simulink model "Bodies_8_Lift_Actuation"  (R2024a)
settings: Solver=ode15s  StartTime=0.0  StopTime=10.0  MaxStep=1e-2  RelTol=1e-3  AbsTol=1e-4  EnableMultiTasking=on
PostLoadFcn:
  | warning off mech2:compiler:topologyAnalysis:DanglingBlock
values from neighbouring files (symbols this model uses):
  rad = 5    [Plot_Extr_Data_Ring_withBoxFillet_forSlide.m]    (also in Plot_Link_Extr_Data_forSlide.m)
undefined symbols (not defined in the file or in its folder): Local, SCL_Par, X, Y, Z
libraries: sm_lib x89, sm_scissor_lift_lib x28, nesl_utility x14, fl_lib x8, sh_lib x4, simulink x1
(part 2 of 4)

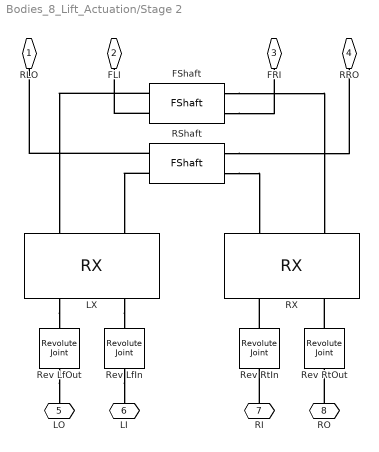
== system Bodies_8_Lift_Actuation/Stage 2 ==
  FShaft : sm_scissor_lift_lib/FShaft  sep_outer_outer=SCL_Par.Link_Sep.Outer_Outer  sep_outer_inner=SCL_Par.Link_Sep.Outer_Inner  shaft_radius=SCL_Par.Trans_Shaft.Radius  shaft_density=SCL_Par.Trans_Shaft.Density  shaft_color=SCL_Par.Trans_Shaft.Color  shaft_opacity=SCL_Par.Trans_Shaft.Opacity
  LX : sm_scissor_lift_lib/RX  leftright=Left  link_length_in=SCL_Par.Link.Length  link_length_out=SCL_Par.Link.Length  link_width_in=SCL_Par.Link.Width  link_width_out=SCL_Par.Link.Width  link_thickness_in=SCL_Par.Link.Thick  link_thickness_out=SCL_Par.Link.Thick  link_hole_radius_in=SCL_Par.Link.HolRad  link_hole_radius_out=SCL_Par.Link.HolRad  link_density_in=SCL_Par.Link.Density  link_density_out=SCL_Par.Link.Density  link_color_in=SCL_Par.Link.ColorI  link_color_out=SCL_Par.Link.ColorO  link_opacity_in=SCL_Par.Link.Opacity  link_opacity_out=SCL_Par.Link.Opacity  shaft_length=SCL_Par.Link_Sep.Outer_Inner  shaft_radius=SCL_Par.Link_Pin.Radius  shaft_density=SCL_Par.Link_Pin.Density  shaft_color=SCL_Par.Link_Pin.Color  shaft_opacity=SCL_Par.Link_Pin.Opacity  imgfile=Crossbar_RX_IMAGE.jpg
  RShaft : sm_scissor_lift_lib/FShaft  sep_outer_outer=SCL_Par.Link_Sep.Outer_Outer  sep_outer_inner=SCL_Par.Link_Sep.Outer_Inner  shaft_radius=SCL_Par.Trans_Shaft.Radius  shaft_density=SCL_Par.Trans_Shaft.Density  shaft_color=SCL_Par.Trans_Shaft.Color  shaft_opacity=SCL_Par.Trans_Shaft.Opacity
  RX : sm_scissor_lift_lib/RX  leftright=Right  link_length_in=SCL_Par.Link.Length  link_length_out=SCL_Par.Link.Length  link_width_in=SCL_Par.Link.Width  link_width_out=SCL_Par.Link.Width  link_thickness_in=SCL_Par.Link.Thick  link_thickness_out=SCL_Par.Link.Thick  link_hole_radius_in=SCL_Par.Link.HolRad  link_hole_radius_out=SCL_Par.Link.HolRad  link_density_in=SCL_Par.Link.Density  link_density_out=SCL_Par.Link.Density  link_color_in=SCL_Par.Link.ColorI  link_color_out=SCL_Par.Link.ColorO  link_opacity_in=SCL_Par.Link.Opacity  link_opacity_out=SCL_Par.Link.Opacity  shaft_length=SCL_Par.Link_Sep.Outer_Inner  shaft_radius=SCL_Par.Link_Pin.Radius  shaft_density=SCL_Par.Link_Pin.Density  shaft_color=SCL_Par.Link_Pin.Color  shaft_opacity=SCL_Par.Link_Pin.Opacity  imgfile=Crossbar_RX_IMAGE.jpg
  Rev LfIn : sm_lib/Joints/Revolute Joint  JointMode=Normal  CompositeWrenchDir=FollowerOnBase  CompositeWrenchFrame=BaseFrame  SenseConstraintForce=off  SenseConstraintTorque=off  SenseTotalForce=off  SenseTotalTorque=off  PositionTargetSpecify=off  PositionTargetPriority=Low  PositionTargetValue=0  PositionTargetValueUnits=deg  VelocityTargetSpecify=off  VelocityTargetPriority=High  VelocityTargetValue=0  VelocityTargetValueUnits=rad/s  EquilibriumPosition=0  EquilibriumPositionUnits=deg  SpringStiffness=0  SpringStiffnessUnits=N*m/rad  DampingCoefficient=0  DampingCoefficientUnits=N*m/(rad/s)  LowerLimitSpecify=off  LowerLimitBound=-90  LowerLimitBoundUnits=deg  LowerLimitStiffness=1e4  LowerLimitStiffnessUnits=N*m/deg  LowerLimitDamping=10  LowerLimitDampingUnits=N*m/(deg/s)  LowerLimitTransitionRegionWidth=0.1  LowerLimitTransitionRegionWidthUnits=deg  UpperLimitSpecify=off  UpperLimitBound=90  UpperLimitBoundUnits=deg  UpperLimitStiffness=1e4  UpperLimitStiffnessUnits=N*m/deg  UpperLimitDamping=10  UpperLimitDampingUnits=N*m/(deg/s)  UpperLimitTransitionRegionWidth=0.1  UpperLimitTransitionRegionWidthUnits=deg  TorqueActuationMode=NoTorque  MotionActuationMode=ComputedMotion  SensePosition=off  SenseVelocity=off  SenseAcceleration=off  SenseTorqueForce=off  SenseLowerLimitTorqueForce=off  SenseUpperLimitTorqueForce=off
  Rev LfOut : sm_lib/Joints/Revolute Joint  JointMode=Normal  CompositeWrenchDir=FollowerOnBase  CompositeWrenchFrame=BaseFrame  SenseConstraintForce=off  SenseConstraintTorque=off  SenseTotalForce=off  SenseTotalTorque=off  PositionTargetSpecify=off  PositionTargetPriority=Low  PositionTargetValue=0  PositionTargetValueUnits=deg  VelocityTargetSpecify=off  VelocityTargetPriority=High  VelocityTargetValue=0  VelocityTargetValueUnits=rad/s  EquilibriumPosition=0  EquilibriumPositionUnits=deg  SpringStiffness=0  SpringStiffnessUnits=N*m/rad  DampingCoefficient=0  DampingCoefficientUnits=N*m/(rad/s)  LowerLimitSpecify=off  LowerLimitBound=-90  LowerLimitBoundUnits=deg  LowerLimitStiffness=1e4  LowerLimitStiffnessUnits=N*m/deg  LowerLimitDamping=10  LowerLimitDampingUnits=N*m/(deg/s)  LowerLimitTransitionRegionWidth=0.1  LowerLimitTransitionRegionWidthUnits=deg  UpperLimitSpecify=off  UpperLimitBound=90  UpperLimitBoundUnits=deg  UpperLimitStiffness=1e4  UpperLimitStiffnessUnits=N*m/deg  UpperLimitDamping=10  UpperLimitDampingUnits=N*m/(deg/s)  UpperLimitTransitionRegionWidth=0.1  UpperLimitTransitionRegionWidthUnits=deg  TorqueActuationMode=NoTorque  MotionActuationMode=ComputedMotion  SensePosition=off  SenseVelocity=off  SenseAcceleration=off  SenseTorqueForce=off  SenseLowerLimitTorqueForce=off  SenseUpperLimitTorqueForce=off
  Rev RtIn : sm_lib/Joints/Revolute Joint  JointMode=Normal  CompositeWrenchDir=FollowerOnBase  CompositeWrenchFrame=BaseFrame  SenseConstraintForce=off  SenseConstraintTorque=off  SenseTotalForce=off  SenseTotalTorque=off  PositionTargetSpecify=on  PositionTargetPriority=High  PositionTargetValue=-2*SCL_Par.Init.Base_Angle  PositionTargetValueUnits=deg  VelocityTargetSpecify=off  VelocityTargetPriority=High  VelocityTargetValue=0  VelocityTargetValueUnits=rad/s  EquilibriumPosition=0  EquilibriumPositionUnits=deg  SpringStiffness=0  SpringStiffnessUnits=N*m/rad  DampingCoefficient=0  DampingCoefficientUnits=N*m/(rad/s)  LowerLimitSpecify=off  LowerLimitBound=-90  LowerLimitBoundUnits=deg  LowerLimitStiffness=1e4  LowerLimitStiffnessUnits=N*m/deg  LowerLimitDamping=10  LowerLimitDampingUnits=N*m/(deg/s)  LowerLimitTransitionRegionWidth=0.1  LowerLimitTransitionRegionWidthUnits=deg  UpperLimitSpecify=off  UpperLimitBound=90  UpperLimitBoundUnits=deg  UpperLimitStiffness=1e4  UpperLimitStiffnessUnits=N*m/deg  UpperLimitDamping=10  UpperLimitDampingUnits=N*m/(deg/s)  UpperLimitTransitionRegionWidth=0.1  UpperLimitTransitionRegionWidthUnits=deg  TorqueActuationMode=NoTorque  MotionActuationMode=ComputedMotion  SensePosition=off  SenseVelocity=off  SenseAcceleration=off  SenseTorqueForce=off  SenseLowerLimitTorqueForce=off  SenseUpperLimitTorqueForce=off
  Rev RtOut : sm_lib/Joints/Revolute Joint  JointMode=Normal  CompositeWrenchDir=FollowerOnBase  CompositeWrenchFrame=BaseFrame  SenseConstraintForce=off  SenseConstraintTorque=off  SenseTotalForce=off  SenseTotalTorque=off  PositionTargetSpecify=off  PositionTargetPriority=Low  PositionTargetValue=0  PositionTargetValueUnits=deg  VelocityTargetSpecify=off  VelocityTargetPriority=High  VelocityTargetValue=0  VelocityTargetValueUnits=rad/s  EquilibriumPosition=0  EquilibriumPositionUnits=deg  SpringStiffness=0  SpringStiffnessUnits=N*m/rad  DampingCoefficient=0  DampingCoefficientUnits=N*m/(rad/s)  LowerLimitSpecify=off  LowerLimitBound=-90  LowerLimitBoundUnits=deg  LowerLimitStiffness=1e4  LowerLimitStiffnessUnits=N*m/deg  LowerLimitDamping=10  LowerLimitDampingUnits=N*m/(deg/s)  LowerLimitTransitionRegionWidth=0.1  LowerLimitTransitionRegionWidthUnits=deg  UpperLimitSpecify=off  UpperLimitBound=90  UpperLimitBoundUnits=deg  UpperLimitStiffness=1e4  UpperLimitStiffnessUnits=N*m/deg  UpperLimitDamping=10  UpperLimitDampingUnits=N*m/(deg/s)  UpperLimitTransitionRegionWidth=0.1  UpperLimitTransitionRegionWidthUnits=deg  TorqueActuationMode=NoTorque  MotionActuationMode=ComputedMotion  SensePosition=off  SenseVelocity=off  SenseAcceleration=off  SenseTorqueForce=off  SenseLowerLimitTorqueForce=off  SenseUpperLimitTorqueForce=off
  RLO : PMIOPort  Side=Left
  FLI : PMIOPort  Port=2  Side=Left
  FRI : PMIOPort  Port=3  Side=Left
  RRO : PMIOPort  Port=4  Side=Left
  LO : PMIOPort  Port=5  Side=Right
  LI : PMIOPort  Port=6  Side=Right
  RI : PMIOPort  Port=7  Side=Right
  RO : PMIOPort  Port=8  Side=Right
  connections:
  Rev LfIn/LConn1 -- LI/RConn1
  Rev LfOut/LConn1 -- LO/RConn1
  LX/RConn2 -- Rev LfIn/RConn1
  LX/RConn1 -- Rev LfOut/RConn1
  RShaft/LConn2 -- LX/LConn2
  RShaft/LConn1 -- RLO/RConn1
  RShaft/RConn1 -- RRO/RConn1
  FShaft/LConn2 -- FLI/RConn1
  FShaft/LConn1 -- LX/LConn1
  FShaft/RConn2 -- FRI/RConn1
  RShaft/RConn2 -- RX/LConn1
  FShaft/RConn1 -- RX/LConn2
  Rev RtIn/RConn1 -- RX/RConn1
  Rev RtOut/RConn1 -- RX/RConn2
  RI/RConn1 -- Rev RtIn/LConn1
  RO/RConn1 -- Rev RtOut/LConn1

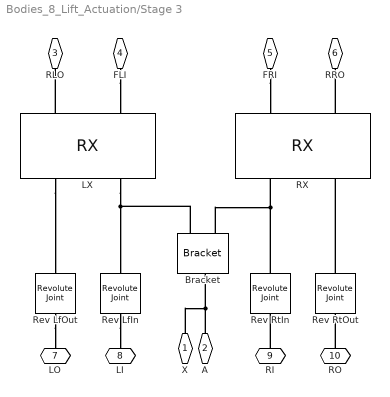
== system Bodies_8_Lift_Actuation/Stage 3 ==
  Bracket : sm_scissor_lift_lib/Bracket  fl_w=SCL_Par.Act.Brkt.Flange.Width  fl_h=SCL_Par.Act.Brkt.Flange.Height  T=SCL_Par.Act.Brkt.Flange.Thickness  w_link=SCL_Par.Link.Width  offset_l=SCL_Par.Act.Brkt.Flange.Offset_L  offset_h=SCL_Par.Act.Brkt.Flange.Offset_H  flupdown=Up  flfrontrear=Front  fl_density=SCL_Par.Act.Brkt.Flange.Density  fl_clr=SCL_Par.Act.Brkt.Flange.Color  fl_opc=SCL_Par.Act.Brkt.Flange.Opacity  shaft_length=SCL_Par.Link_Sep.Outer_Outer-SCL_Par.Link_Sep.Outer_Inner*2  shaft_radius=SCL_Par.Act.Brkt.Shaft.Radius  shaft_density=SCL_Par.Act.Brkt.Shaft.Density  shaft_color=SCL_Par.Act.Brkt.Shaft.Color  shaft_opacity=SCL_Par.Act.Brkt.Shaft.Opacity
  LX : sm_scissor_lift_lib/RX  leftright=Left  link_length_in=SCL_Par.Link.Length  link_length_out=SCL_Par.Link.Length  link_width_in=SCL_Par.Link.Width  link_width_out=SCL_Par.Link.Width  link_thickness_in=SCL_Par.Link.Thick  link_thickness_out=SCL_Par.Link.Thick  link_hole_radius_in=SCL_Par.Link.HolRad  link_hole_radius_out=SCL_Par.Link.HolRad  link_density_in=SCL_Par.Link.Density  link_density_out=SCL_Par.Link.Density  link_color_in=SCL_Par.Link.ColorI  link_color_out=SCL_Par.Link.ColorO  link_opacity_in=SCL_Par.Link.Opacity  link_opacity_out=SCL_Par.Link.Opacity  shaft_length=SCL_Par.Link_Sep.Outer_Inner  shaft_radius=SCL_Par.Link_Pin.Radius  shaft_density=SCL_Par.Link_Pin.Density  shaft_color=SCL_Par.Link_Pin.Color  shaft_opacity=SCL_Par.Link_Pin.Opacity  imgfile=Crossbar_RX_IMAGE.jpg
  RX : sm_scissor_lift_lib/RX  leftright=Right  link_length_in=SCL_Par.Link.Length  link_length_out=SCL_Par.Link.Length  link_width_in=SCL_Par.Link.Width  link_width_out=SCL_Par.Link.Width  link_thickness_in=SCL_Par.Link.Thick  link_thickness_out=SCL_Par.Link.Thick  link_hole_radius_in=SCL_Par.Link.HolRad  link_hole_radius_out=SCL_Par.Link.HolRad  link_density_in=SCL_Par.Link.Density  link_density_out=SCL_Par.Link.Density  link_color_in=SCL_Par.Link.ColorI  link_color_out=SCL_Par.Link.ColorO  link_opacity_in=SCL_Par.Link.Opacity  link_opacity_out=SCL_Par.Link.Opacity  shaft_length=SCL_Par.Link_Sep.Outer_Inner  shaft_radius=SCL_Par.Link_Pin.Radius  shaft_density=SCL_Par.Link_Pin.Density  shaft_color=SCL_Par.Link_Pin.Color  shaft_opacity=SCL_Par.Link_Pin.Opacity  imgfile=Crossbar_RX_IMAGE.jpg
  Rev LfIn : sm_lib/Joints/Revolute Joint  JointMode=Normal  CompositeWrenchDir=FollowerOnBase  CompositeWrenchFrame=BaseFrame  SenseConstraintForce=off  SenseConstraintTorque=off  SenseTotalForce=off  SenseTotalTorque=off  PositionTargetSpecify=off  PositionTargetPriority=Low  PositionTargetValue=0  PositionTargetValueUnits=deg  VelocityTargetSpecify=off  VelocityTargetPriority=High  VelocityTargetValue=0  VelocityTargetValueUnits=rad/s  EquilibriumPosition=0  EquilibriumPositionUnits=deg  SpringStiffness=0  SpringStiffnessUnits=N*m/rad  DampingCoefficient=0  DampingCoefficientUnits=N*m/(rad/s)  LowerLimitSpecify=off  LowerLimitBound=-90  LowerLimitBoundUnits=deg  LowerLimitStiffness=1e4  LowerLimitStiffnessUnits=N*m/deg  LowerLimitDamping=10  LowerLimitDampingUnits=N*m/(deg/s)  LowerLimitTransitionRegionWidth=0.1  LowerLimitTransitionRegionWidthUnits=deg  UpperLimitSpecify=off  UpperLimitBound=90  UpperLimitBoundUnits=deg  UpperLimitStiffness=1e4  UpperLimitStiffnessUnits=N*m/deg  UpperLimitDamping=10  UpperLimitDampingUnits=N*m/(deg/s)  UpperLimitTransitionRegionWidth=0.1  UpperLimitTransitionRegionWidthUnits=deg  TorqueActuationMode=NoTorque  MotionActuationMode=ComputedMotion  SensePosition=off  SenseVelocity=off  SenseAcceleration=off  SenseTorqueForce=off  SenseLowerLimitTorqueForce=off  SenseUpperLimitTorqueForce=off
  Rev LfOut : sm_lib/Joints/Revolute Joint  JointMode=Normal  CompositeWrenchDir=FollowerOnBase  CompositeWrenchFrame=BaseFrame  SenseConstraintForce=off  SenseConstraintTorque=off  SenseTotalForce=off  SenseTotalTorque=off  PositionTargetSpecify=off  PositionTargetPriority=Low  PositionTargetValue=0  PositionTargetValueUnits=deg  VelocityTargetSpecify=off  VelocityTargetPriority=High  VelocityTargetValue=0  VelocityTargetValueUnits=rad/s  EquilibriumPosition=0  EquilibriumPositionUnits=deg  SpringStiffness=0  SpringStiffnessUnits=N*m/rad  DampingCoefficient=0  DampingCoefficientUnits=N*m/(rad/s)  LowerLimitSpecify=off  LowerLimitBound=-90  LowerLimitBoundUnits=deg  LowerLimitStiffness=1e4  LowerLimitStiffnessUnits=N*m/deg  LowerLimitDamping=10  LowerLimitDampingUnits=N*m/(deg/s)  LowerLimitTransitionRegionWidth=0.1  LowerLimitTransitionRegionWidthUnits=deg  UpperLimitSpecify=off  UpperLimitBound=90  UpperLimitBoundUnits=deg  UpperLimitStiffness=1e4  UpperLimitStiffnessUnits=N*m/deg  UpperLimitDamping=10  UpperLimitDampingUnits=N*m/(deg/s)  UpperLimitTransitionRegionWidth=0.1  UpperLimitTransitionRegionWidthUnits=deg  TorqueActuationMode=NoTorque  MotionActuationMode=ComputedMotion  SensePosition=off  SenseVelocity=off  SenseAcceleration=off  SenseTorqueForce=off  SenseLowerLimitTorqueForce=off  SenseUpperLimitTorqueForce=off
  Rev RtIn : sm_lib/Joints/Revolute Joint  JointMode=Normal  CompositeWrenchDir=FollowerOnBase  CompositeWrenchFrame=BaseFrame  SenseConstraintForce=off  SenseConstraintTorque=off  SenseTotalForce=off  SenseTotalTorque=off  PositionTargetSpecify=on  PositionTargetPriority=High  PositionTargetValue=-2*SCL_Par.Init.Base_Angle  PositionTargetValueUnits=deg  VelocityTargetSpecify=off  VelocityTargetPriority=High  VelocityTargetValue=0  VelocityTargetValueUnits=rad/s  EquilibriumPosition=0  EquilibriumPositionUnits=deg  SpringStiffness=0  SpringStiffnessUnits=N*m/rad  DampingCoefficient=0  DampingCoefficientUnits=N*m/(rad/s)  LowerLimitSpecify=off  LowerLimitBound=-90  LowerLimitBoundUnits=deg  LowerLimitStiffness=1e4  LowerLimitStiffnessUnits=N*m/deg  LowerLimitDamping=10  LowerLimitDampingUnits=N*m/(deg/s)  LowerLimitTransitionRegionWidth=0.1  LowerLimitTransitionRegionWidthUnits=deg  UpperLimitSpecify=off  UpperLimitBound=90  UpperLimitBoundUnits=deg  UpperLimitStiffness=1e4  UpperLimitStiffnessUnits=N*m/deg  UpperLimitDamping=10  UpperLimitDampingUnits=N*m/(deg/s)  UpperLimitTransitionRegionWidth=0.1  UpperLimitTransitionRegionWidthUnits=deg  TorqueActuationMode=NoTorque  MotionActuationMode=ComputedMotion  SensePosition=off  SenseVelocity=off  SenseAcceleration=off  SenseTorqueForce=off  SenseLowerLimitTorqueForce=off  SenseUpperLimitTorqueForce=off
  Rev RtOut : sm_lib/Joints/Revolute Joint  JointMode=Normal  CompositeWrenchDir=FollowerOnBase  CompositeWrenchFrame=BaseFrame  SenseConstraintForce=off  SenseConstraintTorque=off  SenseTotalForce=off  SenseTotalTorque=off  PositionTargetSpecify=off  PositionTargetPriority=Low  PositionTargetValue=0  PositionTargetValueUnits=deg  VelocityTargetSpecify=off  VelocityTargetPriority=High  VelocityTargetValue=0  VelocityTargetValueUnits=rad/s  EquilibriumPosition=0  EquilibriumPositionUnits=deg  SpringStiffness=0  SpringStiffnessUnits=N*m/rad  DampingCoefficient=0  DampingCoefficientUnits=N*m/(rad/s)  LowerLimitSpecify=off  LowerLimitBound=-90  LowerLimitBoundUnits=deg  LowerLimitStiffness=1e4  LowerLimitStiffnessUnits=N*m/deg  LowerLimitDamping=10  LowerLimitDampingUnits=N*m/(deg/s)  LowerLimitTransitionRegionWidth=0.1  LowerLimitTransitionRegionWidthUnits=deg  UpperLimitSpecify=off  UpperLimitBound=90  UpperLimitBoundUnits=deg  UpperLimitStiffness=1e4  UpperLimitStiffnessUnits=N*m/deg  UpperLimitDamping=10  UpperLimitDampingUnits=N*m/(deg/s)  UpperLimitTransitionRegionWidth=0.1  UpperLimitTransitionRegionWidthUnits=deg  TorqueActuationMode=NoTorque  MotionActuationMode=ComputedMotion  SensePosition=off  SenseVelocity=off  SenseAcceleration=off  SenseTorqueForce=off  SenseLowerLimitTorqueForce=off  SenseUpperLimitTorqueForce=off
  X : PMIOPort  Side=Left
  A : PMIOPort  Port=2  Side=Right
  RLO : PMIOPort  Port=3  Side=Left
  FLI : PMIOPort  Port=4  Side=Left
  FRI : PMIOPort  Port=5  Side=Left
  RRO : PMIOPort  Port=6  Side=Left
  LO : PMIOPort  Port=7  Side=Right
  LI : PMIOPort  Port=8  Side=Right
  RI : PMIOPort  Port=9  Side=Right
  RO : PMIOPort  Port=10  Side=Right
  connections:
  X/RConn1 -- Bracket/LConn1 -- A/RConn1
  Rev RtIn/RConn1 -- Bracket/RConn2 -- RX/RConn1
  RO/RConn1 -- Rev RtOut/LConn1
  RX/LConn2 -- RRO/RConn1
  FLI/RConn1 -- LX/LConn2
  Rev RtOut/RConn1 -- RX/RConn2
  LX/RConn2 -- Bracket/RConn1 -- Rev LfIn/RConn1
  Rev LfOut/LConn1 -- LO/RConn1
  RI/RConn1 -- Rev RtIn/LConn1
  LX/RConn1 -- Rev LfOut/RConn1
  Rev LfIn/LConn1 -- LI/RConn1
  LX/LConn1 -- RLO/RConn1
  FRI/RConn1 -- RX/LConn1

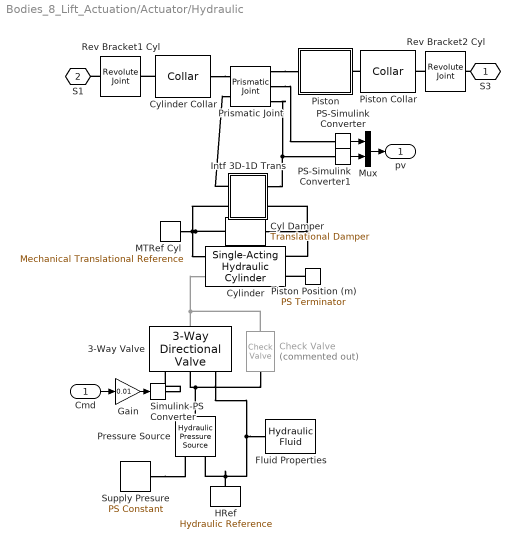
== system Bodies_8_Lift_Actuation/Actuator/Hydraulic ==
  Cmd : Inport
  3-Way Valve : sh_lib/Valves/Directional Valves/3-Way Directional Valve  Tag=Factory Generic  area_spec=1  mdl_type_identical=1  mdl_type_different=1  interp_method_identical=1  interp_method_different=1  extrap_method_identical=1  extrap_method_different=1  A_leak=1e-9 m^2  C_d=0.7  lam_spec=2  B_lam=0.999  Re_cr=12  opening_max=0.01 m  area_max=1e-4*0.1 m^2  opening_max_P_A=0.005 m  area_max_P_A=0.5e-4 m^2  opening_max_A_T=0.005 m  area_max_A_T=0.5e-4 m^2  opening_area_tab="[  -0.002 0 0.005 0.015 ] m"  area_tab="[  1e-12 4e-12 1e-05 1.02e-05 ] m^2"  opening_flow_rate_tab="[  -0.002 0 0.005 0.015 ] m"  pressure_tab="[  -5e+06 -2e+06 2e+06 5e+06 ] Pa"  flow_rate_tab="[  -1e-12 -6e-14 6e+12 1e+11 ; -8e-08 -4e-08 4e+06 8e+06 ; -0.0025 -0.00103 0.001 0.0024 ; -0.00258 -0.001032 0.00106 0.00247 ; ] m^3/s"  opening_area_tab_P_A=[-0.002, 0.0, 0.002, 0.005, 0.015] m  area_tab_P_A=[1.0e-9, 2.0352e-7, 4.0736e-5, 0.00011438, 0.00034356] m^2  opening_flow_rate_tab_P_A=[-0.002, 0.0, 0.002, 0.005, 0.015] m  pressure_tab_P_A=[-10000000.0, -5000000.0, -2000000.0, 2000000.0, 5000000.0, 10000000.0] Pa  flow_rate_tab_P_A=[-1.0e-7, -7.0711e-8, -4.4721e-8, 4.4721e-8, 7.0711e-8, 1.0e-7; -2.0352e-5, -1.4391e-5, -9.1017e-6, 9.1017e-6, 1.4391e-5, 2.0352e-5; -0.0040736, -0.0028805, -0.0018218, 0.0018218, 0.0028805, 0.0040736; -0.011438, -0.0080879, -0.0051152, 0.0051152, 0.0080879, 0.011438; -0.034356, -0.024293, -0.015364, 0.015364, 0.024293, 0.034356] m^3/s  opening_area_tab_A_T=[-0.002, 0.0, 0.002, 0.005, 0.015] m  area_tab_A_T=[1.0e-9, 2.0352e-7, 4.0736e-5, 0.00011438, 0.00034356] m^2  opening_flow_rate_tab_A_T=[-0.002, 0.0, 0.002, 0.005, 0.015] m  pressure_tab_A_T=[-10000000.0, -5000000.0, -2000000.0, 2000000.0, 5000000.0, 10000000.0] Pa  flow_rate_tab_A_T=[-1.0e-7, -7.0711e-8, -4.4721e-8, 4.4721e-8, 7.0711e-8, 1.0e-7; -2.0352e-5, -1.4391e-5, -9.1017e-6, 9.1017e-6, 1.4391e-5, 2.0352e-5; -0.0040736, -0.0028805, -0.0018218, 0.0018218, 0.0028805, 0.0040736; -0.011438, -0.0080879, -0.0051152, 0.0051152, 0.0080879, 0.011438; -0.034356, -0.024293, -0.015364, 0.015364, 0.024293, 0.034356] m^3/s  x_0_P=-0.008 m  x_0_T=-0.008 m
      settings: InternalSimscapePortConfiguration="{\"Bottom\":[],\"Left\":[{\"id\":\"A\",\"label\":\"A\",\"type\":\"foundation.hydraulic.hydraulic\"}],\"Right\":[{\"id\":\"S\",\"label\":\"S\",\"type\":\"input\"},{\"id\":\"P\",\"label\":\"P\",\"type\":\"foundation.hydraulic.hydraulic\"},{\"id\":\"T\",\"label\":\"T\",\"type\":\"foundation.hydraulic.hydraulic\"}],\"Top\":[]}"
  Check Valve : sh_lib/Valves/Directional Valves/Check Valve  Commented=on  area_max=1e-4 m^2  pres_crack=7e6 Pa  pres_max=7.2e6 Pa  C_d=0.7  A_leak=1e-12 m^2  lam_spec=2  B_lam=0.999  Re_cr=12  dynamic=0  tau=0.1 s  area_init=1e-12 m^2
      settings: InternalSimscapePortConfiguration="{\"Bottom\":[],\"Left\":[{\"id\":\"A\",\"label\":\"A\",\"type\":\"foundation.hydraulic.hydraulic\"}],\"Right\":[{\"id\":\"B\",\"label\":\"B\",\"type\":\"foundation.hydraulic.hydraulic\"}],\"Top\":[]}"
  Cyl Damper : fl_lib/Mechanical/Translational Elements/Translational Damper  D=SCL_Par.Act.Spring.Damping*4 N/(m/s)  v_specify=off  v_priority=None  v=0 m/s  v_nominal_specify=off  v_nominal_value=1  v_nominal_unit=m/s  f_specify=off  f_priority=None  f=0 N  f_nominal_specify=off  f_nominal_value=1  f_nominal_unit=N
  Cylinder : sh_lib/Hydraulic Cylinders/Single-Acting Hydraulic Cylinder  Tag=Factory Generic  area=0.002 m^2  stroke=2 m  displacement_spec=foundation.enum.DisplacementSpec.Calculate  init_pos=1 m  dead_vol=1e-06 m^3  init_pressure=0 Pa  k_sh=1.4  stiff=1e+07 N/m  D=250 N/(m/s)  hardstop_model=3  transition=0.1 mm  or=1
      settings: InternalSimscapePortConfiguration="{\"Bottom\":[],\"Left\":[{\"id\":\"C\",\"label\":\"C\",\"type\":\"foundation.mechanical.translational.translational\"},{\"id\":\"A\",\"label\":\"A\",\"type\":\"foundation.hydraulic.hydraulic\"}],\"Right\":[{\"id\":\"R\",\"label\":\"R\",\"type\":\"foundation.mechanical.translational.translational\"},{\"id\":\"P\",\"label\":\"p\",\"type\":\"output\"}],\"Top\":[]}"
  Cylinder Collar : sm_scissor_lift_lib/Collar  collar_length=SCL_Par.Act.Collar.Length  collar_radius=SCL_Par.Act.Collar.Radius  cylinder_length=SCL_Par.Act.Cylinder.Length  cylinder_radius=SCL_Par.Act.Cylinder.Radius  cylinder_ori=Local +Z  material_density=SCL_Par.Act.Collar.Density  material_color=SCL_Par.Act.Collar.Color  material_opacity=SCL_Par.Act.Collar.Opacity
  Fluid Properties : sh_lib/Hydraulic Utilities/Hydraulic Fluid  Tag=Factory Generic  SelFluid=1  SysTemp=40  TrapAir=0.002  ViscDerFactor=1  range_error=2
  Gain : Gain  Gain=0.01
  HRef : fl_lib/Hydraulic/Hydraulic Elements/Hydraulic Reference  Tag=Factory Generic
  Intf 3D-1D Trans : Subsystem
  MTRef Cyl : fl_lib/Mechanical/Translational Elements/Mechanical Translational Reference  Tag=Factory Generic
  Mux : Mux  Inputs=2
  PS-Simulink Converter : nesl_utility/PS-Simulink Converter  PhysicalDomain=network_engine_domain  SubClassName=ps_output  LeftPortType=input  RightPortType=output  PseudoPeriodic=off  Frequencies=[]  VectorFormat=1-D array  Unit=1  AffineConversion=off
  PS-Simulink Converter1 : nesl_utility/PS-Simulink Converter  PhysicalDomain=network_engine_domain  SubClassName=ps_output  LeftPortType=input  RightPortType=output  PseudoPeriodic=off  Frequencies=[]  VectorFormat=1-D array  Unit=1  AffineConversion=off
  Piston : Subsystem
      mask Display: image('Piston_Shaft_IMAGE.jpg');
  Piston Collar : sm_scissor_lift_lib/Collar  collar_length=SCL_Par.Act.Collar.Length  collar_radius=SCL_Par.Act.Collar.Radius  cylinder_length=SCL_Par.Act.Piston_Seat.Length  cylinder_radius=SCL_Par.Act.Piston_Seat.Radius  cylinder_ori=Local -Z  material_density=SCL_Par.Act.Collar.Density  material_color=SCL_Par.Act.Collar.Color  material_opacity=SCL_Par.Act.Collar.Opacity
  Piston Position (m) : fl_lib/Physical Signals/Sinks/PS Terminator
  Pressure Source : fl_lib/Hydraulic/Hydraulic Sources/Hydraulic Pressure Source  Tag=Factory Generic
      settings: InternalSimscapePortConfiguration="{\"Bottom\":[],\"Left\":[{\"id\":\"P\",\"label\":\"P\",\"type\":\"foundation.hydraulic.hydraulic\"}],\"Right\":[{\"id\":\"S\",\"label\":\"S\",\"type\":\"input\"},{\"id\":\"T\",\"label\":\"T\",\"type\":\"foundation.hydraulic.hydraulic\"}],\"Top\":[]}"
  Prismatic Joint : sm_lib/Joints/Prismatic Joint  JointMode=Normal  CompositeWrenchDir=FollowerOnBase  CompositeWrenchFrame=BaseFrame  SenseConstraintForce=off  SenseConstraintTorque=off  SenseTotalForce=off  SenseTotalTorque=off  PositionTargetSpecify=off  PositionTargetPriority=High  PositionTargetValue=0  PositionTargetValueUnits=m  VelocityTargetSpecify=off  VelocityTargetPriority=High  VelocityTargetValue=0  VelocityTargetValueUnits=m/s  EquilibriumPosition=SCL_Par.Act.Spring.Equilibrium_Position*0  EquilibriumPositionUnits=cm  SpringStiffness=SCL_Par.Act.Spring.Stiffness*0  SpringStiffnessUnits=N/m  DampingCoefficient=SCL_Par.Act.Spring.Damping*0  DampingCoefficientUnits=N/(m/s)  LowerLimitSpecify=off  LowerLimitBound=-1  LowerLimitBoundUnits=m  LowerLimitStiffness=1e6  LowerLimitStiffnessUnits=N/m  LowerLimitDamping=1e3  LowerLimitDampingUnits=N/(m/s)  LowerLimitTransitionRegionWidth=1e-4  LowerLimitTransitionRegionWidthUnits=m  UpperLimitSpecify=off  UpperLimitBound=1  UpperLimitBoundUnits=m  UpperLimitStiffness=1e6  UpperLimitStiffnessUnits=N/m  UpperLimitDamping=1e3  UpperLimitDampingUnits=N/(m/s)  UpperLimitTransitionRegionWidth=1e-4  UpperLimitTransitionRegionWidthUnits=m  TorqueActuationMode=InputTorque  MotionActuationMode=ComputedMotion  SensePosition=on  SenseVelocity=on  SenseAcceleration=off  SenseTorqueForce=off  SenseLowerLimitTorqueForce=off  SenseUpperLimitTorqueForce=off
  Rev Bracket1 Cyl : sm_lib/Joints/Revolute Joint  JointMode=Normal  CompositeWrenchDir=FollowerOnBase  CompositeWrenchFrame=BaseFrame  SenseConstraintForce=off  SenseConstraintTorque=off  SenseTotalForce=off  SenseTotalTorque=off  PositionTargetSpecify=off  PositionTargetPriority=High  PositionTargetValue=0  PositionTargetValueUnits=rad  VelocityTargetSpecify=off  VelocityTargetPriority=High  VelocityTargetValue=0  VelocityTargetValueUnits=rad/s  EquilibriumPosition=0  EquilibriumPositionUnits=rad  SpringStiffness=0  SpringStiffnessUnits=N*m/rad  DampingCoefficient=0  DampingCoefficientUnits=N*m/(rad/s)  LowerLimitSpecify=off  LowerLimitBound=-90  LowerLimitBoundUnits=deg  LowerLimitStiffness=1e4  LowerLimitStiffnessUnits=N*m/deg  LowerLimitDamping=10  LowerLimitDampingUnits=N*m/(deg/s)  LowerLimitTransitionRegionWidth=0.1  LowerLimitTransitionRegionWidthUnits=deg  UpperLimitSpecify=off  UpperLimitBound=90  UpperLimitBoundUnits=deg  UpperLimitStiffness=1e4  UpperLimitStiffnessUnits=N*m/deg  UpperLimitDamping=10  UpperLimitDampingUnits=N*m/(deg/s)  UpperLimitTransitionRegionWidth=0.1  UpperLimitTransitionRegionWidthUnits=deg  TorqueActuationMode=NoTorque  MotionActuationMode=ComputedMotion  SensePosition=off  SenseVelocity=off  SenseAcceleration=off  SenseTorqueForce=off  SenseLowerLimitTorqueForce=off  SenseUpperLimitTorqueForce=off
  Rev Bracket2 Cyl : sm_lib/Joints/Revolute Joint  JointMode=Normal  CompositeWrenchDir=FollowerOnBase  CompositeWrenchFrame=BaseFrame  SenseConstraintForce=off  SenseConstraintTorque=off  SenseTotalForce=off  SenseTotalTorque=off  PositionTargetSpecify=off  PositionTargetPriority=High  PositionTargetValue=0  PositionTargetValueUnits=rad  VelocityTargetSpecify=off  VelocityTargetPriority=High  VelocityTargetValue=0  VelocityTargetValueUnits=rad/s  EquilibriumPosition=0  EquilibriumPositionUnits=rad  SpringStiffness=0  SpringStiffnessUnits=N*m/rad  DampingCoefficient=0  DampingCoefficientUnits=N*m/(rad/s)  LowerLimitSpecify=off  LowerLimitBound=-90  LowerLimitBoundUnits=deg  LowerLimitStiffness=1e4  LowerLimitStiffnessUnits=N*m/deg  LowerLimitDamping=10  LowerLimitDampingUnits=N*m/(deg/s)  LowerLimitTransitionRegionWidth=0.1  LowerLimitTransitionRegionWidthUnits=deg  UpperLimitSpecify=off  UpperLimitBound=90  UpperLimitBoundUnits=deg  UpperLimitStiffness=1e4  UpperLimitStiffnessUnits=N*m/deg  UpperLimitDamping=10  UpperLimitDampingUnits=N*m/(deg/s)  UpperLimitTransitionRegionWidth=0.1  UpperLimitTransitionRegionWidthUnits=deg  TorqueActuationMode=NoTorque  MotionActuationMode=ComputedMotion  SensePosition=off  SenseVelocity=off  SenseAcceleration=off  SenseTorqueForce=off  SenseLowerLimitTorqueForce=off  SenseUpperLimitTorqueForce=off
  Simulink-PS Converter : nesl_utility/Simulink-PS Converter  PhysicalDomain=network_engine_domain  SubClassName=ps_input  LeftPortType=input  RightPortType=output  PseudoPeriodic=off  Frequencies=[]  NoiseDistribution=none  NoiseParameters=[]  Unit=m  AffineConversion=off  FilteringAndDerivatives=filter  SimscapeFilterOrder=1  InputFilterTimeConstant=0.005  UdotUserProvided=1
  Supply Presure : fl_lib/Physical Signals/Sources/PS Constant  constant=10e5*8
  S3 : PMIOPort  Side=Right
  S1 : PMIOPort  Port=2  Side=Left
  pv : Outport  VectorParamsAs1DForOutWhenUnconnected=off
  wires:
  Mux/1 -> pv/1
  PS-Simulink Converter1/1 -> Mux/2
  PS-Simulink Converter/1 -> Mux/1
  Cmd/1 -> Gain/1
  Gain/1 -> Simulink-PS Converter/1
  connections:
  Rev Bracket1 Cyl/LConn1 -- S1/RConn1
  S3/RConn1 -- Rev Bracket2 Cyl/LConn1
  Rev Bracket2 Cyl/RConn1 -- Piston Collar/LConn1
  Piston Collar/RConn1 -- Piston/LConn1
  Cylinder Collar/LConn1 -- Rev Bracket1 Cyl/RConn1
  Prismatic Joint/RConn1 -- Piston/RConn1
  Prismatic Joint/RConn2 -- PS-Simulink Converter/LConn1
  Prismatic Joint/RConn3 -- PS-Simulink Converter1/LConn1 -- Intf 3D-1D Trans/LConn1
  Cylinder Collar/RConn1 -- Prismatic Joint/LConn1
  Check Valve/RConn1 -- Cylinder/LConn2 -- 3-Way Valve/LConn1
  Cyl Damper/RConn1 -- MTRef Cyl/LConn1 -- Cylinder/LConn1 -- Intf 3D-1D Trans/RConn2
  3-Way Valve/RConn2 -- Pressure Source/LConn1 -- Check Valve/LConn1
  Intf 3D-1D Trans/LConn2 -- Cyl Damper/LConn1 -- Cylinder/RConn1
  Fluid Properties/RConn1 -- 3-Way Valve/RConn3 -- HRef/LConn1 -- Pressure Source/RConn2
  Simulink-PS Converter/RConn1 -- 3-Way Valve/RConn1
  Supply Presure/RConn1 -- Pressure Source/RConn1
  Piston Position (m)/LConn1 -- Cylinder/RConn2
  Intf 3D-1D Trans/RConn1 -- Prismatic Joint/LConn2

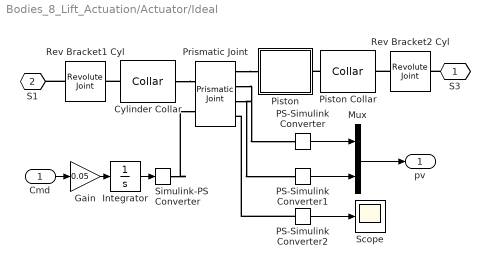
== system Bodies_8_Lift_Actuation/Actuator/Ideal ==
  Cmd : Inport
  Cylinder Collar : sm_scissor_lift_lib/Collar  collar_length=SCL_Par.Act.Collar.Length  collar_radius=SCL_Par.Act.Collar.Radius  cylinder_length=SCL_Par.Act.Cylinder.Length  cylinder_radius=SCL_Par.Act.Cylinder.Radius  cylinder_ori=Local +Z  material_density=SCL_Par.Act.Collar.Density  material_color=SCL_Par.Act.Collar.Color  material_opacity=SCL_Par.Act.Collar.Opacity
  Gain : Gain  Gain=0.05
  Integrator : Integrator  InitialCondition=1.89
  Mux : Mux  Inputs=2
  PS-Simulink Converter : nesl_utility/PS-Simulink Converter  PhysicalDomain=network_engine_domain  SubClassName=ps_output  LeftPortType=input  RightPortType=output  PseudoPeriodic=off  Frequencies=[]  VectorFormat=1-D array  Unit=1  AffineConversion=off
  PS-Simulink Converter1 : nesl_utility/PS-Simulink Converter  PhysicalDomain=network_engine_domain  SubClassName=ps_output  LeftPortType=input  RightPortType=output  PseudoPeriodic=off  Frequencies=[]  VectorFormat=1-D array  Unit=1  AffineConversion=off
  PS-Simulink Converter2 : nesl_utility/PS-Simulink Converter  PhysicalDomain=network_engine_domain  SubClassName=ps_output  LeftPortType=input  RightPortType=output  PseudoPeriodic=off  Frequencies=[]  VectorFormat=1-D array  Unit=1  AffineConversion=off
  Piston : Subsystem
      mask Display: image('Piston_Shaft_IMAGE.jpg');
  Piston Collar : sm_scissor_lift_lib/Collar  collar_length=SCL_Par.Act.Collar.Length  collar_radius=SCL_Par.Act.Collar.Radius  cylinder_length=SCL_Par.Act.Piston_Seat.Length  cylinder_radius=SCL_Par.Act.Piston_Seat.Radius  cylinder_ori=Local -Z  material_density=SCL_Par.Act.Collar.Density  material_color=SCL_Par.Act.Collar.Color  material_opacity=SCL_Par.Act.Collar.Opacity
  Prismatic Joint : sm_lib/Joints/Prismatic Joint  JointMode=Normal  CompositeWrenchDir=FollowerOnBase  CompositeWrenchFrame=BaseFrame  SenseConstraintForce=off  SenseConstraintTorque=off  SenseTotalForce=off  SenseTotalTorque=off  PositionTargetSpecify=off  PositionTargetPriority=High  PositionTargetValue=0  PositionTargetValueUnits=m  VelocityTargetSpecify=off  VelocityTargetPriority=High  VelocityTargetValue=0  VelocityTargetValueUnits=m/s  EquilibriumPosition=SCL_Par.Act.Spring.Equilibrium_Position  EquilibriumPositionUnits=cm  SpringStiffness=SCL_Par.Act.Spring.Stiffness  SpringStiffnessUnits=N/m  DampingCoefficient=SCL_Par.Act.Spring.Damping  DampingCoefficientUnits=N/(m/s)  LowerLimitSpecify=off  LowerLimitBound=-1  LowerLimitBoundUnits=m  LowerLimitStiffness=1e6  LowerLimitStiffnessUnits=N/m  LowerLimitDamping=1e3  LowerLimitDampingUnits=N/(m/s)  LowerLimitTransitionRegionWidth=1e-4  LowerLimitTransitionRegionWidthUnits=m  UpperLimitSpecify=off  UpperLimitBound=1  UpperLimitBoundUnits=m  UpperLimitStiffness=1e6  UpperLimitStiffnessUnits=N/m  UpperLimitDamping=1e3  UpperLimitDampingUnits=N/(m/s)  UpperLimitTransitionRegionWidth=1e-4  UpperLimitTransitionRegionWidthUnits=m  TorqueActuationMode=ComputedTorque  MotionActuationMode=InputMotion  SensePosition=on  SenseVelocity=on  SenseAcceleration=off  SenseTorqueForce=on  SenseLowerLimitTorqueForce=off  SenseUpperLimitTorqueForce=off
  Rev Bracket1 Cyl : sm_lib/Joints/Revolute Joint  JointMode=Normal  CompositeWrenchDir=FollowerOnBase  CompositeWrenchFrame=BaseFrame  SenseConstraintForce=off  SenseConstraintTorque=off  SenseTotalForce=off  SenseTotalTorque=off  PositionTargetSpecify=off  PositionTargetPriority=High  PositionTargetValue=0  PositionTargetValueUnits=rad  VelocityTargetSpecify=off  VelocityTargetPriority=High  VelocityTargetValue=0  VelocityTargetValueUnits=rad/s  EquilibriumPosition=0  EquilibriumPositionUnits=rad  SpringStiffness=0  SpringStiffnessUnits=N*m/rad  DampingCoefficient=0  DampingCoefficientUnits=N*m/(rad/s)  LowerLimitSpecify=off  LowerLimitBound=-90  LowerLimitBoundUnits=deg  LowerLimitStiffness=1e4  LowerLimitStiffnessUnits=N*m/deg  LowerLimitDamping=10  LowerLimitDampingUnits=N*m/(deg/s)  LowerLimitTransitionRegionWidth=0.1  LowerLimitTransitionRegionWidthUnits=deg  UpperLimitSpecify=off  UpperLimitBound=90  UpperLimitBoundUnits=deg  UpperLimitStiffness=1e4  UpperLimitStiffnessUnits=N*m/deg  UpperLimitDamping=10  UpperLimitDampingUnits=N*m/(deg/s)  UpperLimitTransitionRegionWidth=0.1  UpperLimitTransitionRegionWidthUnits=deg  TorqueActuationMode=NoTorque  MotionActuationMode=ComputedMotion  SensePosition=off  SenseVelocity=off  SenseAcceleration=off  SenseTorqueForce=off  SenseLowerLimitTorqueForce=off  SenseUpperLimitTorqueForce=off
  Rev Bracket2 Cyl : sm_lib/Joints/Revolute Joint  JointMode=Normal  CompositeWrenchDir=FollowerOnBase  CompositeWrenchFrame=BaseFrame  SenseConstraintForce=off  SenseConstraintTorque=off  SenseTotalForce=off  SenseTotalTorque=off  PositionTargetSpecify=off  PositionTargetPriority=High  PositionTargetValue=0  PositionTargetValueUnits=rad  VelocityTargetSpecify=off  VelocityTargetPriority=High  VelocityTargetValue=0  VelocityTargetValueUnits=rad/s  EquilibriumPosition=0  EquilibriumPositionUnits=rad  SpringStiffness=0  SpringStiffnessUnits=N*m/rad  DampingCoefficient=0  DampingCoefficientUnits=N*m/(rad/s)  LowerLimitSpecify=off  LowerLimitBound=-90  LowerLimitBoundUnits=deg  LowerLimitStiffness=1e4  LowerLimitStiffnessUnits=N*m/deg  LowerLimitDamping=10  LowerLimitDampingUnits=N*m/(deg/s)  LowerLimitTransitionRegionWidth=0.1  LowerLimitTransitionRegionWidthUnits=deg  UpperLimitSpecify=off  UpperLimitBound=90  UpperLimitBoundUnits=deg  UpperLimitStiffness=1e4  UpperLimitStiffnessUnits=N*m/deg  UpperLimitDamping=10  UpperLimitDampingUnits=N*m/(deg/s)  UpperLimitTransitionRegionWidth=0.1  UpperLimitTransitionRegionWidthUnits=deg  TorqueActuationMode=NoTorque  MotionActuationMode=ComputedMotion  SensePosition=off  SenseVelocity=off  SenseAcceleration=off  SenseTorqueForce=off  SenseLowerLimitTorqueForce=off  SenseUpperLimitTorqueForce=off
  Scope : Scope
  Simulink-PS Converter : nesl_utility/Simulink-PS Converter  PhysicalDomain=network_engine_domain  SubClassName=ps_input  LeftPortType=input  RightPortType=output  PseudoPeriodic=off  Frequencies=[]  NoiseDistribution=none  NoiseParameters=[]  Unit=1  AffineConversion=off  FilteringAndDerivatives=filter  SimscapeFilterOrder=2  InputFilterTimeConstant=0.005  UdotUserProvided=0
  S3 : PMIOPort  Side=Right
  S1 : PMIOPort  Port=2  Side=Left
  pv : Outport  VectorParamsAs1DForOutWhenUnconnected=off
  wires:
  PS-Simulink Converter/1 -> Mux/1
  PS-Simulink Converter1/1 -> Mux/2
  Mux/1 -> pv/1
  Gain/1 -> Integrator/1
  Cmd/1 -> Gain/1
  Integrator/1 -> Simulink-PS Converter/1
  PS-Simulink Converter2/1 -> Scope/1
  connections:
  Cylinder Collar/RConn1 -- Prismatic Joint/LConn1
  Prismatic Joint/RConn3 -- PS-Simulink Converter1/LConn1
  Prismatic Joint/RConn2 -- PS-Simulink Converter/LConn1
  Prismatic Joint/RConn1 -- Piston/RConn1
  Cylinder Collar/LConn1 -- Rev Bracket1 Cyl/RConn1
  Piston Collar/RConn1 -- Piston/LConn1
  Rev Bracket2 Cyl/RConn1 -- Piston Collar/LConn1
  S3/RConn1 -- Rev Bracket2 Cyl/LConn1
  Rev Bracket1 Cyl/LConn1 -- S1/RConn1
  Simulink-PS Converter/RConn1 -- Prismatic Joint/LConn2
  PS-Simulink Converter2/LConn1 -- Prismatic Joint/RConn4

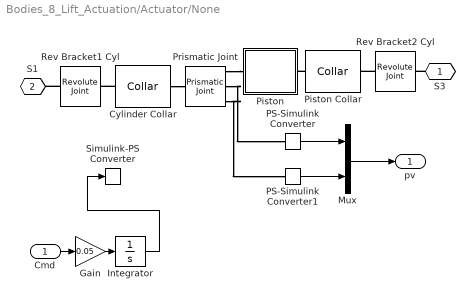
== system Bodies_8_Lift_Actuation/Actuator/None ==
  Cmd : Inport
  Cylinder Collar : sm_scissor_lift_lib/Collar  collar_length=SCL_Par.Act.Collar.Length  collar_radius=SCL_Par.Act.Collar.Radius  cylinder_length=SCL_Par.Act.Cylinder.Length  cylinder_radius=SCL_Par.Act.Cylinder.Radius  cylinder_ori=Local +Z  material_density=SCL_Par.Act.Collar.Density  material_color=SCL_Par.Act.Collar.Color  material_opacity=SCL_Par.Act.Collar.Opacity
  Gain : Gain  Gain=0.05
  Integrator : Integrator  InitialCondition=1.89
  Mux : Mux  Inputs=2
  PS-Simulink Converter : nesl_utility/PS-Simulink Converter  PhysicalDomain=network_engine_domain  SubClassName=ps_output  LeftPortType=input  RightPortType=output  PseudoPeriodic=off  Frequencies=[]  VectorFormat=1-D array  Unit=1  AffineConversion=off
  PS-Simulink Converter1 : nesl_utility/PS-Simulink Converter  PhysicalDomain=network_engine_domain  SubClassName=ps_output  LeftPortType=input  RightPortType=output  PseudoPeriodic=off  Frequencies=[]  VectorFormat=1-D array  Unit=1  AffineConversion=off
  Piston : Subsystem
      mask Display: image('Piston_Shaft_IMAGE.jpg');
  Piston Collar : sm_scissor_lift_lib/Collar  collar_length=SCL_Par.Act.Collar.Length  collar_radius=SCL_Par.Act.Collar.Radius  cylinder_length=SCL_Par.Act.Piston_Seat.Length  cylinder_radius=SCL_Par.Act.Piston_Seat.Radius  cylinder_ori=Local -Z  material_density=SCL_Par.Act.Collar.Density  material_color=SCL_Par.Act.Collar.Color  material_opacity=SCL_Par.Act.Collar.Opacity
  Prismatic Joint : sm_lib/Joints/Prismatic Joint  JointMode=Normal  CompositeWrenchDir=FollowerOnBase  CompositeWrenchFrame=BaseFrame  SenseConstraintForce=off  SenseConstraintTorque=off  SenseTotalForce=off  SenseTotalTorque=off  PositionTargetSpecify=off  PositionTargetPriority=High  PositionTargetValue=0  PositionTargetValueUnits=m  VelocityTargetSpecify=off  VelocityTargetPriority=High  VelocityTargetValue=0  VelocityTargetValueUnits=m/s  EquilibriumPosition=0  EquilibriumPositionUnits=cm  SpringStiffness=0  SpringStiffnessUnits=N/m  DampingCoefficient=0  DampingCoefficientUnits=N/(m/s)  LowerLimitSpecify=off  LowerLimitBound=-1  LowerLimitBoundUnits=m  LowerLimitStiffness=1e6  LowerLimitStiffnessUnits=N/m  LowerLimitDamping=1e3  LowerLimitDampingUnits=N/(m/s)  LowerLimitTransitionRegionWidth=1e-4  LowerLimitTransitionRegionWidthUnits=m  UpperLimitSpecify=off  UpperLimitBound=1  UpperLimitBoundUnits=m  UpperLimitStiffness=1e6  UpperLimitStiffnessUnits=N/m  UpperLimitDamping=1e3  UpperLimitDampingUnits=N/(m/s)  UpperLimitTransitionRegionWidth=1e-4  UpperLimitTransitionRegionWidthUnits=m  TorqueActuationMode=NoTorque  MotionActuationMode=ComputedMotion  SensePosition=on  SenseVelocity=on  SenseAcceleration=off  SenseTorqueForce=off  SenseLowerLimitTorqueForce=off  SenseUpperLimitTorqueForce=off
  Rev Bracket1 Cyl : sm_lib/Joints/Revolute Joint  JointMode=Normal  CompositeWrenchDir=FollowerOnBase  CompositeWrenchFrame=BaseFrame  SenseConstraintForce=off  SenseConstraintTorque=off  SenseTotalForce=off  SenseTotalTorque=off  PositionTargetSpecify=off  PositionTargetPriority=High  PositionTargetValue=0  PositionTargetValueUnits=rad  VelocityTargetSpecify=off  VelocityTargetPriority=High  VelocityTargetValue=0  VelocityTargetValueUnits=rad/s  EquilibriumPosition=0  EquilibriumPositionUnits=rad  SpringStiffness=0  SpringStiffnessUnits=N*m/rad  DampingCoefficient=0  DampingCoefficientUnits=N*m/(rad/s)  LowerLimitSpecify=off  LowerLimitBound=-90  LowerLimitBoundUnits=deg  LowerLimitStiffness=1e4  LowerLimitStiffnessUnits=N*m/deg  LowerLimitDamping=10  LowerLimitDampingUnits=N*m/(deg/s)  LowerLimitTransitionRegionWidth=0.1  LowerLimitTransitionRegionWidthUnits=deg  UpperLimitSpecify=off  UpperLimitBound=90  UpperLimitBoundUnits=deg  UpperLimitStiffness=1e4  UpperLimitStiffnessUnits=N*m/deg  UpperLimitDamping=10  UpperLimitDampingUnits=N*m/(deg/s)  UpperLimitTransitionRegionWidth=0.1  UpperLimitTransitionRegionWidthUnits=deg  TorqueActuationMode=NoTorque  MotionActuationMode=ComputedMotion  SensePosition=off  SenseVelocity=off  SenseAcceleration=off  SenseTorqueForce=off  SenseLowerLimitTorqueForce=off  SenseUpperLimitTorqueForce=off
  Rev Bracket2 Cyl : sm_lib/Joints/Revolute Joint  JointMode=Normal  CompositeWrenchDir=FollowerOnBase  CompositeWrenchFrame=BaseFrame  SenseConstraintForce=off  SenseConstraintTorque=off  SenseTotalForce=off  SenseTotalTorque=off  PositionTargetSpecify=off  PositionTargetPriority=High  PositionTargetValue=0  PositionTargetValueUnits=rad  VelocityTargetSpecify=off  VelocityTargetPriority=High  VelocityTargetValue=0  VelocityTargetValueUnits=rad/s  EquilibriumPosition=0  EquilibriumPositionUnits=rad  SpringStiffness=0  SpringStiffnessUnits=N*m/rad  DampingCoefficient=0  DampingCoefficientUnits=N*m/(rad/s)  LowerLimitSpecify=off  LowerLimitBound=-90  LowerLimitBoundUnits=deg  LowerLimitStiffness=1e4  LowerLimitStiffnessUnits=N*m/deg  LowerLimitDamping=10  LowerLimitDampingUnits=N*m/(deg/s)  LowerLimitTransitionRegionWidth=0.1  LowerLimitTransitionRegionWidthUnits=deg  UpperLimitSpecify=off  UpperLimitBound=90  UpperLimitBoundUnits=deg  UpperLimitStiffness=1e4  UpperLimitStiffnessUnits=N*m/deg  UpperLimitDamping=10  UpperLimitDampingUnits=N*m/(deg/s)  UpperLimitTransitionRegionWidth=0.1  UpperLimitTransitionRegionWidthUnits=deg  TorqueActuationMode=NoTorque  MotionActuationMode=ComputedMotion  SensePosition=off  SenseVelocity=off  SenseAcceleration=off  SenseTorqueForce=off  SenseLowerLimitTorqueForce=off  SenseUpperLimitTorqueForce=off
  Simulink-PS Converter : nesl_utility/Simulink-PS Converter  PhysicalDomain=network_engine_domain  SubClassName=ps_input  LeftPortType=input  RightPortType=output  PseudoPeriodic=off  Frequencies=[]  NoiseDistribution=none  NoiseParameters=[]  Unit=1  AffineConversion=off  FilteringAndDerivatives=filter  SimscapeFilterOrder=2  InputFilterTimeConstant=0.005  UdotUserProvided=0
  S3 : PMIOPort  Side=Right
  S1 : PMIOPort  Port=2  Side=Left
  pv : Outport  VectorParamsAs1DForOutWhenUnconnected=off
  wires:
  Cmd/1 -> Gain/1
  PS-Simulink Converter/1 -> Mux/1
  PS-Simulink Converter1/1 -> Mux/2
  Mux/1 -> pv/1
  Integrator/1 -> Simulink-PS Converter/1
  Gain/1 -> Integrator/1
  connections:
  Cylinder Collar/RConn1 -- Prismatic Joint/LConn1
  Prismatic Joint/RConn3 -- PS-Simulink Converter1/LConn1
  Prismatic Joint/RConn2 -- PS-Simulink Converter/LConn1
  Prismatic Joint/RConn1 -- Piston/RConn1
  Cylinder Collar/LConn1 -- Rev Bracket1 Cyl/RConn1
  Piston Collar/RConn1 -- Piston/LConn1
  Rev Bracket2 Cyl/RConn1 -- Piston Collar/LConn1
  S3/RConn1 -- Rev Bracket2 Cyl/LConn1
  Rev Bracket1 Cyl/LConn1 -- S1/RConn1

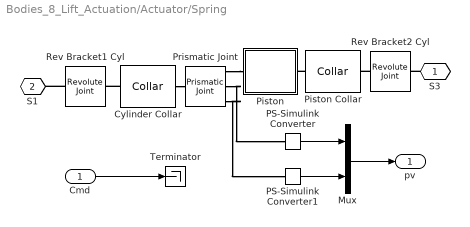
== system Bodies_8_Lift_Actuation/Actuator/Spring ==
  Cmd : Inport
  Cylinder Collar : sm_scissor_lift_lib/Collar  collar_length=SCL_Par.Act.Collar.Length  collar_radius=SCL_Par.Act.Collar.Radius  cylinder_length=SCL_Par.Act.Cylinder.Length  cylinder_radius=SCL_Par.Act.Cylinder.Radius  cylinder_ori=Local +Z  material_density=SCL_Par.Act.Collar.Density  material_color=SCL_Par.Act.Collar.Color  material_opacity=SCL_Par.Act.Collar.Opacity
  Mux : Mux  Inputs=2
  PS-Simulink Converter : nesl_utility/PS-Simulink Converter  PhysicalDomain=network_engine_domain  SubClassName=ps_output  LeftPortType=input  RightPortType=output  PseudoPeriodic=off  Frequencies=[]  VectorFormat=1-D array  Unit=1  AffineConversion=off
  PS-Simulink Converter1 : nesl_utility/PS-Simulink Converter  PhysicalDomain=network_engine_domain  SubClassName=ps_output  LeftPortType=input  RightPortType=output  PseudoPeriodic=off  Frequencies=[]  VectorFormat=1-D array  Unit=1  AffineConversion=off
  Piston : Subsystem
      mask Display: image('Piston_Shaft_IMAGE.jpg');
  Piston Collar : sm_scissor_lift_lib/Collar  collar_length=SCL_Par.Act.Collar.Length  collar_radius=SCL_Par.Act.Collar.Radius  cylinder_length=SCL_Par.Act.Piston_Seat.Length  cylinder_radius=SCL_Par.Act.Piston_Seat.Radius  cylinder_ori=Local -Z  material_density=SCL_Par.Act.Collar.Density  material_color=SCL_Par.Act.Collar.Color  material_opacity=SCL_Par.Act.Collar.Opacity
  Prismatic Joint : sm_lib/Joints/Prismatic Joint  JointMode=Normal  CompositeWrenchDir=FollowerOnBase  CompositeWrenchFrame=BaseFrame  SenseConstraintForce=off  SenseConstraintTorque=off  SenseTotalForce=off  SenseTotalTorque=off  PositionTargetSpecify=off  PositionTargetPriority=High  PositionTargetValue=0  PositionTargetValueUnits=m  VelocityTargetSpecify=off  VelocityTargetPriority=High  VelocityTargetValue=0  VelocityTargetValueUnits=m/s  EquilibriumPosition=SCL_Par.Act.Spring.Equilibrium_Position  EquilibriumPositionUnits=cm  SpringStiffness=SCL_Par.Act.Spring.Stiffness  SpringStiffnessUnits=N/m  DampingCoefficient=SCL_Par.Act.Spring.Damping  DampingCoefficientUnits=N/(m/s)  LowerLimitSpecify=off  LowerLimitBound=-1  LowerLimitBoundUnits=m  LowerLimitStiffness=1e6  LowerLimitStiffnessUnits=N/m  LowerLimitDamping=1e3  LowerLimitDampingUnits=N/(m/s)  LowerLimitTransitionRegionWidth=1e-4  LowerLimitTransitionRegionWidthUnits=m  UpperLimitSpecify=off  UpperLimitBound=1  UpperLimitBoundUnits=m  UpperLimitStiffness=1e6  UpperLimitStiffnessUnits=N/m  UpperLimitDamping=1e3  UpperLimitDampingUnits=N/(m/s)  UpperLimitTransitionRegionWidth=1e-4  UpperLimitTransitionRegionWidthUnits=m  TorqueActuationMode=NoTorque  MotionActuationMode=ComputedMotion  SensePosition=on  SenseVelocity=on  SenseAcceleration=off  SenseTorqueForce=off  SenseLowerLimitTorqueForce=off  SenseUpperLimitTorqueForce=off
  Rev Bracket1 Cyl : sm_lib/Joints/Revolute Joint  JointMode=Normal  CompositeWrenchDir=FollowerOnBase  CompositeWrenchFrame=BaseFrame  SenseConstraintForce=off  SenseConstraintTorque=off  SenseTotalForce=off  SenseTotalTorque=off  PositionTargetSpecify=off  PositionTargetPriority=High  PositionTargetValue=0  PositionTargetValueUnits=rad  VelocityTargetSpecify=off  VelocityTargetPriority=High  VelocityTargetValue=0  VelocityTargetValueUnits=rad/s  EquilibriumPosition=0  EquilibriumPositionUnits=rad  SpringStiffness=0  SpringStiffnessUnits=N*m/rad  DampingCoefficient=0  DampingCoefficientUnits=N*m/(rad/s)  LowerLimitSpecify=off  LowerLimitBound=-90  LowerLimitBoundUnits=deg  LowerLimitStiffness=1e4  LowerLimitStiffnessUnits=N*m/deg  LowerLimitDamping=10  LowerLimitDampingUnits=N*m/(deg/s)  LowerLimitTransitionRegionWidth=0.1  LowerLimitTransitionRegionWidthUnits=deg  UpperLimitSpecify=off  UpperLimitBound=90  UpperLimitBoundUnits=deg  UpperLimitStiffness=1e4  UpperLimitStiffnessUnits=N*m/deg  UpperLimitDamping=10  UpperLimitDampingUnits=N*m/(deg/s)  UpperLimitTransitionRegionWidth=0.1  UpperLimitTransitionRegionWidthUnits=deg  TorqueActuationMode=NoTorque  MotionActuationMode=ComputedMotion  SensePosition=off  SenseVelocity=off  SenseAcceleration=off  SenseTorqueForce=off  SenseLowerLimitTorqueForce=off  SenseUpperLimitTorqueForce=off
  Rev Bracket2 Cyl : sm_lib/Joints/Revolute Joint  JointMode=Normal  CompositeWrenchDir=FollowerOnBase  CompositeWrenchFrame=BaseFrame  SenseConstraintForce=off  SenseConstraintTorque=off  SenseTotalForce=off  SenseTotalTorque=off  PositionTargetSpecify=off  PositionTargetPriority=High  PositionTargetValue=0  PositionTargetValueUnits=rad  VelocityTargetSpecify=off  VelocityTargetPriority=High  VelocityTargetValue=0  VelocityTargetValueUnits=rad/s  EquilibriumPosition=0  EquilibriumPositionUnits=rad  SpringStiffness=0  SpringStiffnessUnits=N*m/rad  DampingCoefficient=0  DampingCoefficientUnits=N*m/(rad/s)  LowerLimitSpecify=off  LowerLimitBound=-90  LowerLimitBoundUnits=deg  LowerLimitStiffness=1e4  LowerLimitStiffnessUnits=N*m/deg  LowerLimitDamping=10  LowerLimitDampingUnits=N*m/(deg/s)  LowerLimitTransitionRegionWidth=0.1  LowerLimitTransitionRegionWidthUnits=deg  UpperLimitSpecify=off  UpperLimitBound=90  UpperLimitBoundUnits=deg  UpperLimitStiffness=1e4  UpperLimitStiffnessUnits=N*m/deg  UpperLimitDamping=10  UpperLimitDampingUnits=N*m/(deg/s)  UpperLimitTransitionRegionWidth=0.1  UpperLimitTransitionRegionWidthUnits=deg  TorqueActuationMode=NoTorque  MotionActuationMode=ComputedMotion  SensePosition=off  SenseVelocity=off  SenseAcceleration=off  SenseTorqueForce=off  SenseLowerLimitTorqueForce=off  SenseUpperLimitTorqueForce=off
  Terminator : Terminator
  S3 : PMIOPort  Side=Right
  S1 : PMIOPort  Port=2  Side=Left
  pv : Outport  VectorParamsAs1DForOutWhenUnconnected=off
  wires:
  Mux/1 -> pv/1
  PS-Simulink Converter1/1 -> Mux/2
  PS-Simulink Converter/1 -> Mux/1
  Cmd/1 -> Terminator/1
  connections:
  Rev Bracket1 Cyl/LConn1 -- S1/RConn1
  S3/RConn1 -- Rev Bracket2 Cyl/LConn1
  Rev Bracket2 Cyl/RConn1 -- Piston Collar/LConn1
  Piston Collar/RConn1 -- Piston/LConn1
  Cylinder Collar/LConn1 -- Rev Bracket1 Cyl/RConn1
  Prismatic Joint/RConn1 -- Piston/RConn1
  Prismatic Joint/RConn2 -- PS-Simulink Converter/LConn1
  Prismatic Joint/RConn3 -- PS-Simulink Converter1/LConn1
  Cylinder Collar/RConn1 -- Prismatic Joint/LConn1
